simulink model "ft_formation_control"  (R2020a)
settings: Solver=VariableStepAuto  StartTime=0.0  StopTime=T  RelTol=1e-3
undefined symbols (not defined in the file or in its folder): params
settings Model: Creator=gaeta  LastModifiedBy=gaeta

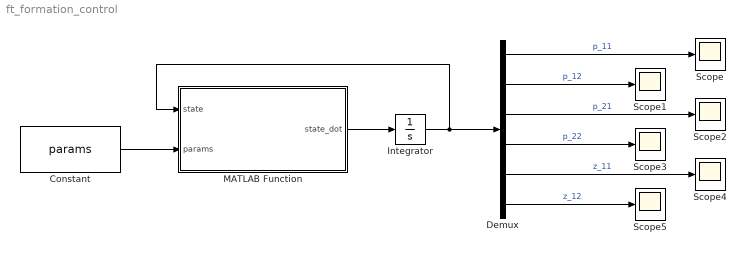
== system ft_formation_control ==
  Constant : Constant  Value=params  OutDataTypeStr=Bus: params_bus
  Demux : Demux  Outputs=6
  Integrator : Integrator
  MATLAB Function : MATLAB Function  TreatAsAtomicUnit=on
  Scope{,1..5} (6 alike) : Scope
  wires:
  MATLAB Function/1(state_dot) -> Integrator/1
  Integrator/1 -> Demux/1, MATLAB Function/1(state)
  Constant/1 -> MATLAB Function/2(params)
  Demux/1 -> Scope/1  "p_11"
  Demux/2 -> Scope1/1  "p_12"
  Demux/3 -> Scope2/1  "p_21"
  Demux/4 -> Scope3/1  "p_22"
  Demux/5 -> Scope4/1  "z_11"
  Demux/6 -> Scope5/1  "z_12"

== matlab function ft_formation_control/MATLAB Function ==
  data: state input size=6; state_dot output size=6; params input
function state_dot = closed_loop(state,params)
%% data
% the state is given by p11 p12 p21 p22 z11 z12 where pi1 and pi2 are the x
% and y momentum of the i-th agent and zi1 and zi2 are the x and y
% component of the distance on the i-th edge
p=state(1:4);
z=state(5:6);
% N=params.N; % agents number
z_star=params.z_star; % desired formation distance
K_c_i=params.K_c; % spring constant

%% physical coeffs 
d=params.d; % friction coeff
d_c=params.d_c; % damping coeffs 
m=params.m; % mass
D_a_i=diag([d d]); % frict. matrix for a single agent
M_i=diag([m m]); % inertia matrix for asingle agent
B=[1 1]'; % incidence matrix
D_c_i=diag([d_c d_c]); % damping matrix

%% closed loop system
D_a=blkdiag(D_a_i,D_a_i);
D_c=(D_c_i);
B_cl=kron(B,eye(2));
M=blkdiag(M_i,M_i);
K_c=K_c_i;

p_dot=[-(D_a+B_cl*D_c*B_cl'), -B_cl]*[M^-1*p; K_c*(z-z_star)];
z_dot=B_cl'*M^-1*p;

state_dot=[p_dot; z_dot];
